simulink model "State_Flow_D"  (R2017a)
settings: Solver=FixedStepDiscrete  StartTime=0.0  StopTime=inf  FixedStep=0.001  RelTol=1e-3  EnableMultiTasking=on
libraries: xpcethercatlib x35, simulink x11, commutil2 x2
(part 2 of 3)

== system State_Flow_D/Out asse B Vite/Fungo ==
  In1 : Inport
  Constant : Constant  Value=0
  Data Type Conversion14 : DataTypeConversion
  Display10 : Display
  EtherCAT PDO Receive9 : xpcethercatlib/EtherCAT PDO Receive  Priority=2  sig_name=Beckoff.Channel 1.Input  sig_offset=0  sig_type=boolean  type_size=1  sig_dim=1  device_id=0  sample_time=0.001000
      settings: SourceProductName=Simulink Real-Time  SourceProductBaseCode=XP
  MATLAB Function : MATLAB Function  TreatAsAtomicUnit=on
  Memory : Memory
  Switch1 : Switch  Criteria=u2 ~= 0  Threshold=2
  Out1 : Outport
  wires:
  EtherCAT PDO Receive9/1 -> Data Type Conversion14/1
  Data Type Conversion14/1 -> MATLAB Function/2(old), Display10/1
  MATLAB Function/1(y) -> Memory/1
  In1/1 -> Switch1/3
  Memory/1 -> Switch1/2, MATLAB Function/1(now)
  Constant/1 -> Switch1/1
  Switch1/1 -> Out1/1

== system State_Flow_D/Sistema Braccia Linea/Velocita vite  ==
  EtherCAT PDO Receive14 : xpcethercatlib/EtherCAT PDO Receive  Priority=2  sig_name=AZ1.Transmit PDO 1.Axis A Actual motor velocity  sig_offset=48  sig_type=int32  type_size=32  sig_dim=1  device_id=0  sample_time=0.001000
      settings: SourceProductName=Simulink Real-Time  SourceProductBaseCode=XP
  EtherCAT PDO Receive15 : xpcethercatlib/EtherCAT PDO Receive  Priority=2  sig_name=AZ1.Transmit PDO 2.Axis B Actual motor velocity  sig_offset=136  sig_type=int32  type_size=32  sig_dim=1  device_id=0  sample_time=0.001000
      settings: SourceProductName=Simulink Real-Time  SourceProductBaseCode=XP
  Vel Asse A conv : MATLAB Function  TreatAsAtomicUnit=on
  Vel Asse B conv : MATLAB Function  TreatAsAtomicUnit=on
  Velocity A : DataTypeConversion
  Velocity B : DataTypeConversion
  Asse A : Outport
  Asse B : Outport  Port=2
  wires:
  EtherCAT PDO Receive15/1 -> Velocity B/1
  EtherCAT PDO Receive14/1 -> Velocity A/1
  Vel Asse A conv/1(vel_A_conv) -> Asse A/1
  Velocity B/1 -> Vel Asse B conv/1(p)
  Vel Asse B conv/1(vel_B_conv) -> Asse B/1
  Velocity A/1 -> Vel Asse A conv/1(vA)

== system State_Flow_D/Sistema Vite/Actual A ==
  Pos : Inport
  Offset : Inport  Port=2
  Rif asse B : Inport  Port=3
  Discrete Derivative A : simulink/Discrete/Discrete Derivative  gainval=1.0  ICPrevScaledInput=0.0  OutMin=[]  OutMax=[]  OutDataType=fixdt(1, 16)  OutScaling=2^-10  DoSatur=off
  Display31 : Display
  Posizione attuale Vite A : Subsystem
  Sum : Sum  Inputs=|-+
  A attuale : Outport
  wires:
  Offset/1 -> Sum/1
  Posizione attuale Vite A/1(A Att) -> A attuale/1, Discrete Derivative A/1
  Sum/1 -> Posizione attuale Vite A/1(Comp Vite A)
  Rif asse B/1 -> Posizione attuale Vite A/2("Comp Vite B ")
  Pos/1 -> Sum/2
  Discrete Derivative A/1 -> Display31/1

== system State_Flow_D/Sistema Vite/Clock reale ==
  cr : Inport
  offset : Inport  Port=2
  Sum2 : Sum  Inputs=-+|
  Ck : Outport
  wires:
  Sum2/1 -> Ck/1
  offset/1 -> Sum2/1
  cr/1 -> Sum2/2

== system State_Flow_D/Sistema Vite/Coppia VIte A finale ==
  Pos : Inport
  Vel : Inport  Port=2
  Gain : Gain  Gain=300*1000/0.36
  Gain6 : Gain  Gain=7.5*1000/0.36
  Sum9 : Sum  Inputs=|++
  Coppia : Outport
  wires:
  Pos/1 -> Gain/1
  Sum9/1 -> Coppia/1
  Gain6/1 -> Sum9/2
  Vel/1 -> Gain6/1
  Gain/1 -> Sum9/1

== system State_Flow_D/Sistema Vite/Velocita vite  ==
  EtherCAT PDO Receive14 : xpcethercatlib/EtherCAT PDO Receive  Priority=2  sig_name=AZ2.Transmit PDO 1.Axis A Actual motor velocity  sig_offset=304  sig_type=int32  type_size=32  sig_dim=1  device_id=0  sample_time=0.001000
      settings: SourceProductName=Simulink Real-Time  SourceProductBaseCode=XP
  EtherCAT PDO Receive15 : xpcethercatlib/EtherCAT PDO Receive  Priority=2  sig_name=AZ2.Transmit PDO 2.Axis B Actual motor velocity  sig_offset=392  sig_type=int32  type_size=32  sig_dim=1  device_id=0  sample_time=0.001000
      settings: SourceProductName=Simulink Real-Time  SourceProductBaseCode=XP
  Vel Asse A conv : MATLAB Function  TreatAsAtomicUnit=on
  Vel Asse B conv : MATLAB Function  TreatAsAtomicUnit=on
  Velocity A : DataTypeConversion
  Velocity B : DataTypeConversion
  Asse A : Outport
  Asse B : Outport  Port=2
  wires:
  EtherCAT PDO Receive15/1 -> Velocity B/1
  EtherCAT PDO Receive14/1 -> Velocity A/1
  Vel Asse A conv/1(vel_A_conv) -> Asse A/1
  Velocity B/1 -> Vel Asse B conv/1(p), Vel Asse A conv/2(vB)
  Vel Asse B conv/1(vel_B_conv) -> Asse B/1
  Velocity A/1 -> Vel Asse A conv/1(vA)

== system State_Flow_D/Sistema Vite/Actual A/Posizione attuale Vite A ==
  Comp Vite A : Inport
  "Comp Vite B " : Inport  Port=2
  Asse A conv : MATLAB Function  TreatAsAtomicUnit=on
  Asse B conv v : MATLAB Function  TreatAsAtomicUnit=on
  Sum5 : Sum
  A Att : Outport
  wires:
  Asse A conv/1(pos_A_conv) -> Sum5/1
  Asse B conv v/1(pos_B_conv_v) -> Sum5/2
  Comp Vite A/1 -> Asse A conv/1(p)
  Sum5/1 -> A Att/1
  "Comp Vite B "/1 -> Asse B conv v/1(p)

== matlab function State_Flow_D/Movimento Braccia/Cinematica Inversa1 ==
  data: x0old input; y0old input; theta1_0 input; theta2_0 input; time input; x0 output; y0 output
function [x0, y0] = fcn(x0old, y0old, theta1_0, theta2_0, time)

if time == 0 

d = 0.09; 
l = 0.25;

A = l^2*(sin(theta2_0)-sin(theta1_0))^2 + (-2*d -l*(cos(theta2_0)-cos(theta1_0)))^2;
B = -2*l^2*d*(sin(theta2_0)-sin(theta1_0))*(cos(theta2_0)+cos(theta1_0)) + ...
    l*(sin(theta2_0)-sin(theta1_0))*(-2*d -l*(cos(theta2_0)-cos(theta1_0)))*(-2*d -2*l*cos(theta2_0)) - ...
    2*l*sin(theta2_0)*(-2*d -l*(cos(theta2_0)-cos(theta1_0)))^2;
C = l^2*d^2*(cos(theta2_0)+cos(theta1_0))^2 -l*d*(cos(theta2_0)+cos(theta1_0))*(-2*d -l*(cos(theta2_0)-cos(theta1_0)))*(-2*d -2*l*cos(theta2_0)) + ...
    (d^2 + 2*d*l*cos(theta2_0))*(-2*d - l*(cos(theta2_0)-cos(theta1_0)))^2;

% Posizione Y end-effector
y0 = (-B + sqrt(B^2 - 4*A*C))/(2*A);
% Posizione X end-effector
x0 = (y0*l*(sin(theta2_0)-sin(theta1_0)) - l*d*(cos(theta2_0)+cos(theta1_0)))/(-2*d -l*(cos(theta2_0)-cos(theta1_0)));
else 
    x0 = x0old;
    y0 = y0old;
end

== matlab function State_Flow_D/Movimento Braccia/MATLAB Function ==
  data: x input; xp output; y input; yp output; bool input
function [xp,yp] = fcn(x, y, bool)
if bool == 4
    xp = x;
    yp = y;
else
    xp = 0;
    yp = 0;
end

== matlab function State_Flow_D/Sistema Braccia Linea/Velocita vite /Vel Asse A conv ==
  data: vA input; vel_A_conv output
function vel_A_conv = fcn(vA)
vel_A_conv = (vA)  *(2*pi)/163840/64;

== matlab function State_Flow_D/Sistema Braccia Linea/Velocita vite /Vel Asse B conv ==
  data: p input; vel_B_conv output
function vel_B_conv = fcn(p)
vel_B_conv = p  *(2*pi)/163840/64;

== matlab function State_Flow_D/Sistema Vite/Actual A/Posizione attuale Vite A/Asse A conv ==
  data: p input; pos_A_conv output
function pos_A_conv = fcn(p)
pos_A_conv = p * 0.02/(2*pi) * pi/2048/40;

== matlab function State_Flow_D/Sistema Vite/Rifermento Asse A Vite ==
  data: t input; ldm_pos output; h input; T input; ldm_vel output
function [ldm_pos, ldm_vel] = fcn(t,h,T)

xv = 0.3;
 x = t/T;
Ca=1/(xv*(1-xv));
Cv = 1/(1-xv);

if( x>= 0 && x < xv)
    f = Ca;
    F = Ca*x;
    G= Ca*x^2/2;
elseif(x >= xv && x < (1-xv) )
    f = 0;
    F = Cv;
    G= Ca*xv^2/2 + Cv*(x-xv);
elseif( x >= (1-xv) && x <= 1 )
    f = -Ca;
    xloc = x-(1-xv);
    F = Cv -Ca*xloc;
    G= Ca*xv^2/2 + Cv*(1-2*xv) + Cv*xloc -Ca*xloc^2/2;
else
    f=0;
    F=0;
    G= Ca*xv^2/2 + Cv*(1-2*xv) + Cv*xv -Ca*xv^2/2;
end

ldm_pos = G*h;
ldm_vel = F*h/T;

== matlab function State_Flow_D/LED Status/MATLAB Function ==
  data: u input; y output
function y = fcn(u)
if u == 2 ||u == 3
    y = 1;
else
    y = 0;
end

== matlab function State_Flow_D/LED Status/MATLAB Function1 ==
  data: u input; y output
function y = fcn(u)
if u == 1 || u == 2 || u == 4
    y = 1;
else
    y = 0;
end

== matlab function State_Flow_D/LED Status/MATLAB Function2 ==
  data: u input; y output
function y = fcn(u)
if u == 4 || u == 5
    y = 1;
else
    y = 0;
end

== matlab function State_Flow_D/Sistema Vite/Asse B conv ==
  data: p input; pos_B_conv output
function pos_B_conv = fcn(p)
pos_B_conv = p * pi/2048/40;

== matlab function State_Flow_D/Sistema Vite/Asse B ==
  data: t input; ldm_pos output; h input; T input; ldm_vel output
function [ldm_pos, ldm_vel] = fcn(t,h,T)

xv = 0.3;
 x = t/T;
Ca=1/(xv*(1-xv));
Cv = 1/(1-xv);

if( x>= 0 && x < xv)
    f = Ca;
    F = Ca*x;
    G= Ca*x^2/2;
elseif(x >= xv && x < (1-xv) )
    f = 0;
    F = Cv;
    G= Ca*xv^2/2 + Cv*(x-xv);
elseif( x >= (1-xv) && x <= 1 )
    f = -Ca;
    xloc = x-(1-xv);
    F = Cv -Ca*xloc;
    G= Ca*xv^2/2 + Cv*(1-2*xv) + Cv*xloc -Ca*xloc^2/2;
else
    f=0;
    F=0;
    G= Ca*xv^2/2 + Cv*(1-2*xv) + Cv*xv -Ca*xv^2/2;
end

ldm_pos = G*h;
ldm_vel = F*h/T;

== matlab function State_Flow_D/Sistema Vite/Actual A/Posizione attuale Vite A/Asse B conv v ==
  data: p input; pos_B_conv_v output
function pos_B_conv_v = fcn(p)
pos_B_conv_v = p * 0.02/(2*pi) * pi/2048/40;

== matlab function State_Flow_D/Sistema Vite/Velocita vite /Vel Asse A conv ==
  data: vA input; vel_A_conv output; vB input
function vel_A_conv = fcn(vA, vB)
vel_A_conv = (vA+vB) * 0.02/(2*pi) * pi/20480/40;

== matlab function State_Flow_D/Sistema Vite/Velocita vite /Vel Asse B conv ==
  data: p input; vel_B_conv output
function vel_B_conv = fcn(p)
vel_B_conv = p  * pi/20480/40;

== stateflow chart State_Flow_D/State flow robot ==
  settings: sampleTime=0.001
  state Step1
    entry:
    Bool = 0;
  state Step2
    entry:
    CoppiaH = 0;
  state Posizionamento
    state OffSet
      entry:
      CoppiaH = 0;
      CoppiaA = 0;
      CoppiaB = 0;
      OffA = posA;
      OffB = posB;
      OffA_0 = posA;
      OffB_0 = posB;
      Bool = 2;
      Luci = 3;
    state SetA
      entry:
      CoppiaA = 0;
      C1 = 0;
    state SetB1
      entry:
      CoppiaB = 0;
      C2 = 0;
    state Discesa_Vite
      entry:
      OffA_vite = posA_vite;
      CoppiaH=700;
    state SetB
      entry:
      CoppiaB = 0;
      C2 = 0;
    state SetA1
      entry:
      CoppiaA = 0;
      C1 = 0;
    Discesa_Vite -> OffSet : [posA_vite - OffA_vite >= 0.038/conv_vite]
    SetB1 -> Discesa_Vite : [C2 == 0]
    SetA -> SetB1 : [posB - OffB_0 >= 40*pi/180/conv]
    SetA1 -> Discesa_Vite : [C1 == 0]
    SetB -> SetA1 : [posA - OffA_0 >= 110*pi/180/conv]
  state Traiettoria
    entry:
    OffT = Clock;
    OffA_vite = posA_vite;
    OffB_vite = posB_vite;
    Luci = 4;
    Bool = 4;
  state Stop
    entry:
    Bool = 5;
    Luci = 5;
  state Coppie
    entry:
    OffA_0 = posA;
    OffB_0 = posB;
    CoppiaA = 1250;
    CoppiaB = 1250;
    CoppiaH = 0;
    Luci = 2;
  state Home
    entry:
    [CoppiaA, CoppiaB, CoppiaH] = Homing(fc, fcA, fcB);
    Bool = 1;
    conv =  (2*pi)/16384/64;
    conv_vite = 0.02/(2*pi) * pi/2048/40;
    Luci = 1;
    C1 = 1;
    C2 = 1;
    H = 0;
  state Step3
    entry:
    CoppiaA = 0;
    CoppiaB = 0;
  state [CA,CB,CH] = Homing(fc,fcA,fcB) [function]
  (default) -> Step1
  Coppie -> SetA [order 1] : [posA - OffA_0 >= 110*pi/180/conv]
  Step1 -> Home : [Status==1079]
  Step2 -> Coppie : [fcA == 1 && fcB==1]
  Home -> Step2 [order 2] : [fc==0]
  Traiettoria -> Stop : after(60,sec)
  OffSet -> Traiettoria
  Coppie -> SetB [order 2] : [posB - OffB_0 >= 40*pi/180/conv]
  Step3 -> Coppie : [fc==0]
  Home -> Step3 [order 1] : [fcA==1 && fcB==1]
  data: fc function_input double size=1; CA function_output; CB function_output; CH function_output; fcA function_input double size=1; fcB function_input double size=1; Clock input; posA_vite input; posB_vite input; SampleTime constant double; Status input; fc input; posA input; posB input; Bool output; OffT output; CoppiaH output; OffA_vite output; OffB_vite output; OffA output; OffB output; CoppiaA output; CoppiaB output; fcA input; fcB input; conv local; Luci output; OffA_0 local; OffB_0 local; C1 local; C2 local; conv_vite local; velA input; velB input; H output

== matlab function State_Flow_D/Movimento Braccia/Cinematica Inversa ==
  data: x input; theta1 output; y input; theta2 output
function [theta1, theta2] = fcn(x, y)

d = 0.09; 
l = 0.25;

p = 2*d*l + 2*x*l;
e = 2*y*l;
f = x^2 + d^2 + y^2 + 2*x*d;
a = -2*d*l + 2*x*l;
b = +2*y*l;
c = x^2 + d^2 + y^2 - 2*x*d;



   theta1 = 2*atan2(e + sqrt(p^2 + e^2 -f^2), p +f);


   theta2 = 2*atan2(b - sqrt(a^2 + b^2 -c^2), a +c);
   if (theta2) < -deg2rad(200)
       theta2 = theta2 + 2*pi;
   end

== matlab function State_Flow_D/Movimento Braccia/Asse B conv brac1 ==
  data: p input; pos_B_conv output
function pos_B_conv = fcn(p)
pos_B_conv = p * (2*pi)/16384/64;

== matlab function State_Flow_D/State flow robot/Homing/MATLAB Function ==
  data: fc input; CA output; fcA input; fcB input; CB output; CH output
function [CA, CB, CH] = fcn(fc, fcA, fcB)

CA = -1250;
CB = -1250;
CH = -600;

if fc < 1
    CH = 0;
end
if fcA == 1
    CA = 0;
end
if fcB == 1
    CB = 0;
end

== matlab function State_Flow_D/Out asse A Vite/Fungo/MATLAB Function ==
  data: now input; old input; y output
function y = fcn(now, old)
if old == 0 && now == 1
    y = 1;
else
    y = old;
end

== matlab function State_Flow_D/Out asse B Vite/Fungo/MATLAB Function ==
  data: now input; old input; y output
function y = fcn(now, old)
if old == 0 && now == 1
    y = 1;
else
    y = old;
end

== matlab function State_Flow_D/Out Asse A Braccia/Fungo/MATLAB Function ==
  data: now input; old input; y output
function y = fcn(now, old)
if old == 0 && now == 1
    y = 1;
else
    y = old;
end

== matlab function State_Flow_D/Out Asse B Braccia/Fungo/MATLAB Function ==
  data: now input; old input; y output
function y = fcn(now, old)
if old == 0 && now == 1
    y = 1;
else
    y = old;
end

== matlab function State_Flow_D/Velocita vite /Vel Asse A conv ==
  data: vA input; vel_A_conv output
function vel_A_conv = fcn(vA)
vel_A_conv = (vA)  *(2*pi)/163840/64;

== matlab function State_Flow_D/Velocita vite /Vel Asse B conv ==
  data: p input; vel_B_conv output
function vel_B_conv = fcn(p)
vel_B_conv = p  *(2*pi)/163840/64;

== matlab function State_Flow_D/Sistema Braccia Linea/Asse A conv bracc2 ==
  data: p input; pos_A_conv output
function pos_A_conv = fcn(p)
pos_A_conv = p * (2*pi)/16384/64;

== matlab function State_Flow_D/Sistema Braccia Linea/Asse B conv brac1 ==
  data: p input; pos_B_conv output
function pos_B_conv = fcn(p)
pos_B_conv = p * (2*pi)/16384/64;

== matlab function State_Flow_D/Sistema Braccia Linea/Cinematica Inversa ==
  data: x input; theta1 output; y input; theta2 output
function [theta1, theta2] = fcn(x, y)

d = 0.09; 
l = 0.25;

p = 2*d*l + 2*x*l;
e = 2*y*l;
f = x^2 + d^2 + y^2 + 2*x*d;
a = -2*d*l + 2*x*l;
b = +2*y*l;
c = x^2 + d^2 + y^2 - 2*x*d;



   theta1 = 2*atan2(e + sqrt(p^2 + e^2 -f^2), p +f);


   theta2 = 2*atan2(b - sqrt(a^2 + b^2 -c^2), a +c);
   if (theta2) < -deg2rad(200)
       theta2 = theta2 + 2*pi;
   end

== matlab function State_Flow_D/Sistema Braccia Linea/Cinematica Inversa vel ==
  data: theta1 input; theta2 input; x input; y input; xp input; theta1_p output; yp input; theta2_p output
function [theta1_p, theta2_p] = fcn(theta1, theta2,x, y, xp, yp)

d = 0.09; 
l = 0.25;

N21 = -l*sin(theta1)*(x+d-l*cos(theta1)) + l*cos(theta1)*(y-l*sin(theta1));

N22 = -l*cos(theta2)*(y-l*sin(theta2))*(x+d-l*cos(theta1))/(x-d-l*cos(theta2)) + l*sin(theta2)*(x+d-l*cos(theta1));

D2 = y-l*sin(theta1) - (y-l*sin(theta2))*(x+d-l*cos(theta1))/(x-d-l*cos(theta2));

J21 = N21/D2;

J22 = N22/D2;

J11 = -(y-l*sin(theta2))/(x-d-l*cos(theta2))*(J21);

J12 = -(y-l*sin(theta2))/(x-d-l*cos(theta2))*(J22) -l*sin(theta2) + (y-l*sin(theta2))/(x-d-l*cos(theta2))*(l*cos(theta2));

J = [J11 J12; J21 J22];

theta_p = J^-1 * [xp; yp];
theta1_p = theta_p(1);
theta2_p = theta_p(2);

== matlab function State_Flow_D/Sistema Braccia Linea/Cinematica Inversa1 ==
  data: theta1_0 input; x0 output; theta2_0 input; y0 output
function [x0, y0] = fcn(theta1_0, theta2_0)

d = 0.09; 
l = 0.25;

A = l^2*(sin(theta2_0)-sin(theta1_0))^2 + (-2*d -l*(cos(theta2_0)-cos(theta1_0)))^2;
B = -2*l^2*d*(sin(theta2_0)-sin(theta1_0))*(cos(theta2_0)+cos(theta1_0)) + ...
    l*(sin(theta2_0)-sin(theta1_0))*(-2*d -l*(cos(theta2_0)-cos(theta1_0)))*(-2*d -2*l*cos(theta2_0)) - ...
    2*l*sin(theta2_0)*(-2*d -l*(cos(theta2_0)-cos(theta1_0)))^2;
C = l^2*d^2*(cos(theta2_0)+cos(theta1_0))^2 -l*d*(cos(theta2_0)+cos(theta1_0))*(-2*d -l*(cos(theta2_0)-cos(theta1_0)))*(-2*d -2*l*cos(theta2_0)) + ...
    (d^2 + 2*d*l*cos(theta2_0))*(-2*d - l*(cos(theta2_0)-cos(theta1_0)))^2;

% Posizione Y end-effector
y0 = (-B + sqrt(B^2 - 4*A*C))/(2*A)
% Posizione X end-effector
x0 = (y0*l*(sin(theta2_0)-sin(theta1_0)) - l*d*(cos(theta2_0)+cos(theta1_0)))/(-2*d -l*(cos(theta2_0)-cos(theta1_0)))

== matlab function State_Flow_D/Sistema Braccia Linea/x ==
  data: t input; ldm_pos output; h input; T input; ldm_vel output
function [ldm_pos, ldm_vel] = fcn(t,h,T)

xv = 0.3;
 x = t/T;
Ca=1/(xv*(1-xv));
Cv = 1/(1-xv);

if( x>= 0 && x < xv)
    f = Ca;
    F = Ca*x;
    G= Ca*x^2/2;
elseif(x >= xv && x < (1-xv) )
    f = 0;
    F = Cv;
    G= Ca*xv^2/2 + Cv*(x-xv);
elseif( x >= (1-xv) && x <= 1 )
    f = -Ca;
    xloc = x-(1-xv);
    F = Cv -Ca*xloc;
    G= Ca*xv^2/2 + Cv*(1-2*xv) + Cv*xloc -Ca*xloc^2/2;
else
    f=0;
    F=0;
    G= Ca*xv^2/2 + Cv*(1-2*xv) + Cv*xv -Ca*xv^2/2;
end

ldm_pos = G*h;
ldm_vel = F*h/T;

== matlab function State_Flow_D/Sistema Braccia Linea/y ==
  data: t input; ldm_pos output; h input; T input; ldm_vel output
function [ldm_pos, ldm_vel] = fcn(t,h,T)

xv = 0.3;
 x = t/T;
Ca=1/(xv*(1-xv));
Cv = 1/(1-xv);

if( x>= 0 && x < xv)
    f = Ca;
    F = Ca*x;
    G= Ca*x^2/2;
elseif(x >= xv && x < (1-xv) )
    f = 0;
    F = Cv;
    G= Ca*xv^2/2 + Cv*(x-xv);
elseif( x >= (1-xv) && x <= 1 )
    f = -Ca;
    xloc = x-(1-xv);
    F = Cv -Ca*xloc;
    G= Ca*xv^2/2 + Cv*(1-2*xv) + Cv*xloc -Ca*xloc^2/2;
else
    f=0;
    F=0;
    G= 1;
end

ldm_pos = G*h;
ldm_vel = F*h/T;

== matlab function State_Flow_D/Movimento Braccia/Asse A conv brac ==
  data: p input; pos_A_conv output
function pos_A_conv = fcn(p)
pos_A_conv = p * (2*pi)/16384/64;

== matlab function State_Flow_D/Movimento Braccia/Subsystem/Cerchio ==
  data: xc output; t input; yc output; T input; r input; xc_p output; yc_p output
function [xc, yc, xc_p, yc_p] = fcn(t, T, r)
xv = 0.4;
xj = 0.1;
x = t/T;
Ca = 1/((1-xv)*(xv-xj));
if ( x >= 0 && x < xj)            %acc crescente positiva
    f = Ca/xj*x;
    F = (1/2)*Ca/xj*x^2;
    G = (1/6)*Ca/xj*x^3;
    J = Ca/xj;

  elseif (x >= xj && x < (xv-xj))   %acc costante positiva
    f = Ca;
    F = Ca*x - (1/2)*Ca*xj;
    G = (1/2)*Ca*x^2 - (1/2)*Ca*xj*x + (1/6)*Ca*xj^2;
    J = 0;

  elseif( x>= (xv-xj) && x < xv)    %acc decrescente positiva
    f = -Ca/xj*x + Ca*xv/xj;
    F = -(1/2)*Ca/xj*x^2 + Ca/xj*xv*x - Ca*(xj + (1/2)/xj*xv^2 - xv);
    G = -(1/6)*Ca/xj*x^3 + (1/2)*Ca/xj*xv*x^2 - Ca*(xj + (1/2)/xj*xv^2 - xv)*x ...
        - (1/2)*Ca*xv^2  + (1/6)*Ca/xj*xv^3 + (1/2)*Ca*xv*xj;
    J = -Ca/xj;

  elseif( x>= xv && x < (1-xv))     %acc costante nulla
    f = 0;
    F = Ca*(xv - xj);
    G = Ca*(xv - xj)*x - (1/2)*Ca*xv^2 + (1/2)*Ca*xv*xj;
    J = 0;
    
  elseif( x>= (1-xv) && x < (1-xv+xj))   %acc decrescente negativa
    f = -Ca/xj*x + Ca/xj*(1-xv);
    F = -(1/2)*Ca/xj*x^2 + Ca/xj*(1-xv)*x + Ca*(xv-xj) - (1/2)*Ca/xj*(1-xv)^2;
    G = -(1/6)*Ca/xj*x^3 + (1/2)*Ca/xj*(1-xv)*x^2 + Ca*(xv-xj)*x - (1/2)*Ca/xj*(1-xv)^2*x ...
        - (1/2)*Ca*xv^2 + (1/2)*Ca*xv*xj + (1/6)*Ca/xj*(1-xv)^3;
    J = -Ca/xj;
    
  elseif( x>= (1-xv+xj) && x < (1-xj))   %acc costante negativa
    f = -Ca; 
    F = -Ca*x + Ca - (1/2)*Ca*xj;
    G = -(1/2)*Ca*x^2 + Ca*x - (1/2)*Ca*xj*x + 1 - Ca*(-(1/2)*xj + (1/6)*xj^2 + (1/2));
    J = 0;
    
  elseif( x>= (1-xj) && x <= 1)          %acc crescente negativa
    f = Ca/xj*(x-1);
    F = (1/2)*Ca/xj*x^2 - Ca/xj*x +(1/2)*Ca/xj;
    G = (1/6)*Ca/xj*x^3 - (1/2)*Ca/xj*x^2 +(1/2)*Ca/xj*x + 1 - (1/6)*Ca/xj;
    J = Ca/xj;
    
  else                                   %acc costante nulla
    f = 0;
    F = 0;
    G = 1;
    J = 0;
end
  
 alfa = G*2*pi;
 alfa_p = F*2*pi/T;
 xc = r*cos(pi/2-alfa);
 yc = r*sin(pi/2-alfa) - r;
 xc_p = r*sin(pi/2-alfa)*alfa_p;
 yc_p = -r*cos(pi/2-alfa)*alfa_p;

== matlab function State_Flow_D/Movimento Braccia/Subsystem/Quadrato ==
  data: xq output; yq output; t input; T input; h input; xq_p output; yq_p output
function [xq, yq, xq_p, yq_p] = fcn(t, T, h)
xv = 0.4;
xj = 0.1;
x1 = t/(0.5*T/4);
x2 = (t-0.5*T/4)/(T/4);
x3 = (t-1.5*T/4)/(T/4);
x4 = (t-2.5*T/4)/(T/4);
x5 = (t-3.5*T/4)/(0.5*T/4);
Ca = 1/((1-xv)*(xv-xj));
% Ca = 1/(xv*(1-xv));
% Cv = 1/(1-xv);


if t > 0 && t <= 0.5*T/4
  
  if ( x1 >= 0 && x1 < xj)            %acc crescente positiva
    f = Ca/xj*x1;
    F = (1/2)*Ca/xj*x1^2;
    G = (1/6)*Ca/xj*x1^3;
    J = Ca/xj;

  elseif (x1 >= xj && x1 < (xv-xj))   %acc costante positiva
    f = Ca;
    F = Ca*x1 - (1/2)*Ca*xj;
    G = (1/2)*Ca*x1^2 - (1/2)*Ca*xj*x1 + (1/6)*Ca*xj^2;
    J = 0;

  elseif( x1>= (xv-xj) && x1 < xv)    %acc decrescente positiva
    f = -Ca/xj*x1 + Ca*xv/xj;
    F = -(1/2)*Ca/xj*x1^2 + Ca/xj*xv*x1 - Ca*(xj + (1/2)/xj*xv^2 - xv);
    G = -(1/6)*Ca/xj*x1^3 + (1/2)*Ca/xj*xv*x1^2 - Ca*(xj + (1/2)/xj*xv^2 - xv)*x1 ...
        - (1/2)*Ca*xv^2  + (1/6)*Ca/xj*xv^3 + (1/2)*Ca*xv*xj;
    J = -Ca/xj;

  elseif( x1>= xv && x1 < (1-xv))     %acc costante nulla
    f = 0;
    F = Ca*(xv - xj);
    G = Ca*(xv - xj)*x1 - (1/2)*Ca*xv^2 + (1/2)*Ca*xv*xj;
    J = 0;
    
  elseif( x1>= (1-xv) && x1 < (1-xv+xj))   %acc decrescente negativa
    f = -Ca/xj*x1 + Ca/xj*(1-xv);
    F = -(1/2)*Ca/xj*x1^2 + Ca/xj*(1-xv)*x1 + Ca*(xv-xj) - (1/2)*Ca/xj*(1-xv)^2;
    G = -(1/6)*Ca/xj*x1^3 + (1/2)*Ca/xj*(1-xv)*x1^2 + Ca*(xv-xj)*x1 - (1/2)*Ca/xj*(1-xv)^2*x1 ...
        - (1/2)*Ca*xv^2 + (1/2)*Ca*xv*xj + (1/6)*Ca/xj*(1-xv)^3;
    J = -Ca/xj;
    
  elseif( x1>= (1-xv+xj) && x1 < (1-xj))   %acc costante negativa
    f = -Ca; 
    F = -Ca*x1 + Ca - (1/2)*Ca*xj;
    G = -(1/2)*Ca*x1^2 + Ca*x1 - (1/2)*Ca*xj*x1 + 1 - Ca*(-(1/2)*xj + (1/6)*xj^2 + (1/2));
    J = 0;
    
  elseif( x1>= (1-xj) && x1 <= 1)          %acc crescente negativa
    f = Ca/xj*(x1-1);
    F = (1/2)*Ca/xj*x1^2 - Ca/xj*x1 +(1/2)*Ca/xj;
    G = (1/6)*Ca/xj*x1^3 - (1/2)*Ca/xj*x1^2 +(1/2)*Ca/xj*x1 + 1 - (1/6)*Ca/xj;
    J = Ca/xj;
    
  else                                   %acc costante nulla
    f = 0;
    F = 0;
    G = 1;
    J = 0;
  end
    xq = G*h/2;
    xq_p = F*(h/2)/(T/4);
    yq = 0;
    yq_p = 0; 

elseif t > 0.5*T/4 && t <= 1.5*T/4
    Ca = 1/((1-xv)*(xv-xj));
% Cj = Ca/xj;
  
  if ( x2 >= 0 && x2 < xj)            %acc crescente positiva
    f = Ca/xj*x2;
    F = (1/2)*Ca/xj*x2^2;
    G = (1/6)*Ca/xj*x2^3;
    J = Ca/xj;

  elseif (x2 >= xj && x2 < (xv-xj))   %acc costante positiva
    f = Ca;
    F = Ca*x2 - (1/2)*Ca*xj;
    G = (1/2)*Ca*x2^2 - (1/2)*Ca*xj*x2 + (1/6)*Ca*xj^2;
    J = 0;

  elseif( x2>= (xv-xj) && x2 < xv)    %acc decrescente positiva
    f = -Ca/xj*x2 + Ca*xv/xj;
    F = -(1/2)*Ca/xj*x2^2 + Ca/xj*xv*x2 - Ca*(xj + (1/2)/xj*xv^2 - xv);
    G = -(1/6)*Ca/xj*x2^3 + (1/2)*Ca/xj*xv*x2^2 - Ca*(xj + (1/2)/xj*xv^2 - xv)*x2 ...
        - (1/2)*Ca*xv^2  + (1/6)*Ca/xj*xv^3 + (1/2)*Ca*xv*xj;
    J = -Ca/xj;

  elseif( x2>= xv && x2 < (1-xv))     %acc costante nulla
    f = 0;
    F = Ca*(xv - xj);
    G = Ca*(xv - xj)*x2 - (1/2)*Ca*xv^2 + (1/2)*Ca*xv*xj;
    J = 0;
    
  elseif( x2>= (1-xv) && x2 < (1-xv+xj))   %acc decrescente negativa
    f = -Ca/xj*x2 + Ca/xj*(1-xv);
    F = -(1/2)*Ca/xj*x2^2 + Ca/xj*(1-xv)*x2 + Ca*(xv-xj) - (1/2)*Ca/xj*(1-xv)^2;
    G = -(1/6)*Ca/xj*x2^3 + (1/2)*Ca/xj*(1-xv)*x2^2 + Ca*(xv-xj)*x2 - (1/2)*Ca/xj*(1-xv)^2*x2 ...
        - (1/2)*Ca*xv^2 + (1/2)*Ca*xv*xj + (1/6)*Ca/xj*(1-xv)^3;
    J = -Ca/xj;
    
  elseif( x2>= (1-xv+xj) && x2 < (1-xj))   %acc costante negativa
    f = -Ca; 
    F = -Ca*x2 + Ca - (1/2)*Ca*xj;
    G = -(1/2)*Ca*x2^2 + Ca*x2 - (1/2)*Ca*xj*x2 + 1 - Ca*(-(1/2)*xj + (1/6)*xj^2 + (1/2));
    J = 0;
    
  elseif( x2>= (1-xj) && x2 <= 1)          %acc crescente negativa
    f = Ca/xj*(x2-1);
    F = (1/2)*Ca/xj*x2^2 - Ca/xj*x2 +(1/2)*Ca/xj;
    G = (1/6)*Ca/xj*x2^3 - (1/2)*Ca/xj*x2^2 +(1/2)*Ca/xj*x2 + 1 - (1/6)*Ca/xj;
    J = Ca/xj;
    
  else                                   %acc costante nulla
    f = 0;
    F = 0;
    G = 1;
    J = 0;
  end
    xq = h/2;
    xq_p = 0;
    yq = -G*h; 
    yq_p = -F*h/(T/4); 

elseif t > 1.5*T/4 && t <= 2.5*T/4
     Ca = 1/((1-xv)*(xv-xj));
% Cj = Ca/xj;
  
  if ( x3 >= 0 && x3 < xj)            %acc crescente positiva
    f = Ca/xj*x3;
    F = (1/2)*Ca/xj*x3^2;
    G = (1/6)*Ca/xj*x3^3;
    J = Ca/xj;

  elseif (x3 >= xj && x3 < (xv-xj))   %acc costante positiva
    f = Ca;
    F = Ca*x3 - (1/2)*Ca*xj;
    G = (1/2)*Ca*x3^2 - (1/2)*Ca*xj*x3 + (1/6)*Ca*xj^2;
    J = 0;

  elseif( x3>= (xv-xj) && x3 < xv)    %acc decrescente positiva
    f = -Ca/xj*x3 + Ca*xv/xj;
    F = -(1/2)*Ca/xj*x3^2 + Ca/xj*xv*x3 - Ca*(xj + (1/2)/xj*xv^2 - xv);
    G = -(1/6)*Ca/xj*x3^3 + (1/2)*Ca/xj*xv*x3^2 - Ca*(xj + (1/2)/xj*xv^2 - xv)*x3 ...
        - (1/2)*Ca*xv^2  + (1/6)*Ca/xj*xv^3 + (1/2)*Ca*xv*xj;
    J = -Ca/xj;

  elseif( x3>= xv && x3 < (1-xv))     %acc costante nulla
    f = 0;
    F = Ca*(xv - xj);
    G = Ca*(xv - xj)*x3 - (1/2)*Ca*xv^2 + (1/2)*Ca*xv*xj;
    J = 0;
    
  elseif( x3>= (1-xv) && x3 < (1-xv+xj))   %acc decrescente negativa
    f = -Ca/xj*x3 + Ca/xj*(1-xv);
    F = -(1/2)*Ca/xj*x3^2 + Ca/xj*(1-xv)*x3 + Ca*(xv-xj) - (1/2)*Ca/xj*(1-xv)^2;
    G = -(1/6)*Ca/xj*x3^3 + (1/2)*Ca/xj*(1-xv)*x3^2 + Ca*(xv-xj)*x3 - (1/2)*Ca/xj*(1-xv)^2*x3 ...
        - (1/2)*Ca*xv^2 + (1/2)*Ca*xv*xj + (1/6)*Ca/xj*(1-xv)^3;
    J = -Ca/xj;
    
  elseif( x3>= (1-xv+xj) && x3 < (1-xj))   %acc costante negativa
    f = -Ca; 
    F = -Ca*x3 + Ca - (1/2)*Ca*xj;
    G = -(1/2)*Ca*x3^2 + Ca*x3 - (1/2)*Ca*xj*x3 + 1 - Ca*(-(1/2)*xj + (1/6)*xj^2 + (1/2));
    J = 0;
    
  elseif( x3>= (1-xj) && x3 <= 1)          %acc crescente negativa
    f = Ca/xj*(x3-1);
    F = (1/2)*Ca/xj*x3^2 - Ca/xj*x3 +(1/2)*Ca/xj;
    G = (1/6)*Ca/xj*x3^3 - (1/2)*Ca/xj*x3^2 +(1/2)*Ca/xj*x3 + 1 - (1/6)*Ca/xj;
    J = Ca/xj;
    
  else                                   %acc costante nulla
    f = 0;
    F = 0;
    G = 1;
    J = 0;
  end
    xq = h/2-G*h;
    xq_p = -F*h/(T/4);
    yq = -h; 
    yq_p = 0; 
 
elseif t > 2.5*T/4 && t <= 3.5*T/4
   Ca = 1/((1-xv)*(xv-xj));
% Cj = Ca/xj;
  
  if ( x4 >= 0 && x4 < xj)            %acc crescente positiva
    f = Ca/xj*x4;
    F = (1/2)*Ca/xj*x4^2;
    G = (1/6)*Ca/xj*x4^3;
    J = Ca/xj;

  elseif (x4 >= xj && x4 < (xv-xj))   %acc costante positiva
    f = Ca;
    F = Ca*x4 - (1/2)*Ca*xj;
    G = (1/2)*Ca*x4^2 - (1/2)*Ca*xj*x4 + (1/6)*Ca*xj^2;
    J = 0;

  elseif( x4>= (xv-xj) && x4 < xv)    %acc decrescente positiva
    f = -Ca/xj*x4 + Ca*xv/xj;
    F = -(1/2)*Ca/xj*x4^2 + Ca/xj*xv*x4 - Ca*(xj + (1/2)/xj*xv^2 - xv);
    G = -(1/6)*Ca/xj*x4^3 + (1/2)*Ca/xj*xv*x4^2 - Ca*(xj + (1/2)/xj*xv^2 - xv)*x4 ...
        - (1/2)*Ca*xv^2  + (1/6)*Ca/xj*xv^3 + (1/2)*Ca*xv*xj;
    J = -Ca/xj;

  elseif( x4>= xv && x4 < (1-xv))     %acc costante nulla
    f = 0;
    F = Ca*(xv - xj);
    G = Ca*(xv - xj)*x4 - (1/2)*Ca*xv^2 + (1/2)*Ca*xv*xj;
    J = 0;
    
  elseif( x4>= (1-xv) && x4 < (1-xv+xj))   %acc decrescente negativa
    f = -Ca/xj*x4 + Ca/xj*(1-xv);
    F = -(1/2)*Ca/xj*x4^2 + Ca/xj*(1-xv)*x4 + Ca*(xv-xj) - (1/2)*Ca/xj*(1-xv)^2;
    G = -(1/6)*Ca/xj*x4^3 + (1/2)*Ca/xj*(1-xv)*x4^2 + Ca*(xv-xj)*x4 - (1/2)*Ca/xj*(1-xv)^2*x4 ...
        - (1/2)*Ca*xv^2 + (1/2)*Ca*xv*xj + (1/6)*Ca/xj*(1-xv)^3;
    J = -Ca/xj;
    
  elseif( x4>= (1-xv+xj) && x4 < (1-xj))   %acc costante negativa
    f = -Ca; 
    F = -Ca*x4 + Ca - (1/2)*Ca*xj;
    G = -(1/2)*Ca*x4^2 + Ca*x4 - (1/2)*Ca*xj*x4 + 1 - Ca*(-(1/2)*xj + (1/6)*xj^2 + (1/2));
    J = 0;
    
  elseif( x4>= (1-xj) && x4 <= 1)          %acc crescente negativa
    f = Ca/xj*(x4-1);
    F = (1/2)*Ca/xj*x4^2 - Ca/xj*x4 +(1/2)*Ca/xj;
    G = (1/6)*Ca/xj*x4^3 - (1/2)*Ca/xj*x4^2 +(1/2)*Ca/xj*x4 + 1 - (1/6)*Ca/xj;
    J = Ca/xj;
    
  else                                   %acc costante nulla
    f = 0;
    F = 0;
    G = 1;
    J = 0;
  end
    xq = -h/2;
    xq_p = 0;
    yq = -h + G*h;
    yq_p = F*h/(T/4); 

elseif t > 3.5*T/4 && t <= 4*T/4
   Ca = 1/((1-xv)*(xv-xj));
% Cj = Ca/xj;
  
  if ( x5 >= 0 && x5 < xj)            %acc crescente positiva
    f = Ca/xj*x5;
    F = (1/2)*Ca/xj*x5^2;
    G = (1/6)*Ca/xj*x5^3;
    J = Ca/xj;

  elseif (x5 >= xj && x5 < (xv-xj))   %acc costante positiva
    f = Ca;
    F = Ca*x5 - (1/2)*Ca*xj;
    G = (1/2)*Ca*x5^2 - (1/2)*Ca*xj*x5 + (1/6)*Ca*xj^2;
    J = 0;

  elseif( x5>= (xv-xj) && x5 < xv)    %acc decrescente positiva
    f = -Ca/xj*x5 + Ca*xv/xj;
    F = -(1/2)*Ca/xj*x5^2 + Ca/xj*xv*x5 - Ca*(xj + (1/2)/xj*xv^2 - xv);
    G = -(1/6)*Ca/xj*x5^3 + (1/2)*Ca/xj*xv*x5^2 - Ca*(xj + (1/2)/xj*xv^2 - xv)*x5 ...
        - (1/2)*Ca*xv^2  + (1/6)*Ca/xj*xv^3 + (1/2)*Ca*xv*xj;
    J = -Ca/xj;

  elseif( x5>= xv && x5 < (1-xv))     %acc costante nulla
    f = 0;
    F = Ca*(xv - xj);
    G = Ca*(xv - xj)*x5 - (1/2)*Ca*xv^2 + (1/2)*Ca*xv*xj;
    J = 0;
    
  elseif( x5>= (1-xv) && x5 < (1-xv+xj))   %acc decrescente negativa
    f = -Ca/xj*x5 + Ca/xj*(1-xv);
    F = -(1/2)*Ca/xj*x5^2 + Ca/xj*(1-xv)*x5 + Ca*(xv-xj) - (1/2)*Ca/xj*(1-xv)^2;
    G = -(1/6)*Ca/xj*x5^3 + (1/2)*Ca/xj*(1-xv)*x5^2 + Ca*(xv-xj)*x5 - (1/2)*Ca/xj*(1-xv)^2*x5 ...
        - (1/2)*Ca*xv^2 + (1/2)*Ca*xv*xj + (1/6)*Ca/xj*(1-xv)^3;
    J = -Ca/xj;
    
  elseif( x5>= (1-xv+xj) && x5 < (1-xj))   %acc costante negativa
    f = -Ca; 
    F = -Ca*x5 + Ca - (1/2)*Ca*xj;
    G = -(1/2)*Ca*x5^2 + Ca*x5 - (1/2)*Ca*xj*x5 + 1 - Ca*(-(1/2)*xj + (1/6)*xj^2 + (1/2));
    J = 0;
    
  elseif( x5>= (1-xj) && x5 <= 1)          %acc crescente negativa
    f = Ca/xj*(x5-1);
    F = (1/2)*Ca/xj*x5^2 - Ca/xj*x5 +(1/2)*Ca/xj;
    G = (1/6)*Ca/xj*x5^3 - (1/2)*Ca/xj*x5^2 +(1/2)*Ca/xj*x5 + 1 - (1/6)*Ca/xj;
    J = Ca/xj;
    
  else                                   %acc costante nulla
    f = 0;
    F = 0;
    G = 1;
    J = 0;
  end
    xq = -h/2 + G*h/2;
    xq_p = F*h/2/(T/4);
    yq = 0
    yq_p = 0; 
else
xq = 0;
yq = 0;
xq_p = 0;
yq_p = 0; 
end

== matlab function State_Flow_D/Movimento Braccia/Quadrato1 ==
  data: x output; t input; y output; T input; h input
function [x, y] = fcn(t, T, h)
X1 = linspace(0, h, 1000*T/4);
X2 = linspace(h, 0, 1000*T/4);
Y1 = linspace(0, -h, 1000*T/4);
Y2 = linspace(-h, 0, 1000*T/4);

if t > 0 && t <= T/4
    y = 0;
    x = X1(t*1000);
elseif t > T/4 && t <= 2*T/4
    x = h;
    y = Y1((t-T/4)*1000);
elseif t > 2*T/4 && t <= 3*T/4
    y = -h;
    x = X2((t-2*T/4)*1000);
elseif t > 3*T/4 && t <= 4*T/4
    x = 0;
    y = Y2((t-3*T/4)*1000);
else
x = 0;
y = 0;
end

== matlab function State_Flow_D/Movimento Braccia/Cinematica Inversa vel ==
  data: theta1 input; theta2 input; x input; y input; xp input; theta1_p output; yp input; theta2_p output
function [theta1_p, theta2_p] = fcn(theta1, theta2,x, y, xp, yp)

d = 0.09; 
l = 0.25;

N21 = -l*sin(theta1)*(x+d-l*cos(theta1)) + l*cos(theta1)*(y-l*sin(theta1));

N22 = -l*cos(theta2)*(y-l*sin(theta2))*(x+d-l*cos(theta1))/(x-d-l*cos(theta2)) + l*sin(theta2)*(x+d-l*cos(theta1));

D2 = y-l*sin(theta1) - (y-l*sin(theta2))*(x+d-l*cos(theta1))/(x-d-l*cos(theta2));

J21 = N21/D2;

J22 = N22/D2;

J11 = -(y-l*sin(theta2))/(x-d-l*cos(theta2))*(J21);

J12 = -(y-l*sin(theta2))/(x-d-l*cos(theta2))*(J22) -l*sin(theta2) + (y-l*sin(theta2))/(x-d-l*cos(theta2))*(l*cos(theta2));

J = [J11 J12; J21 J22];

theta_p = J^-1 * [xp; yp];
theta1_p = theta_p(1);
theta2_p = theta_p(2);

== matlab function State_Flow_D/Movimento Braccia/Velocita vite /Vel Asse A conv ==
  data: vA input; vel_A_conv output
function vel_A_conv = fcn(vA)
vel_A_conv = (vA)  *(2*pi)/163840/64;

== matlab function State_Flow_D/Movimento Braccia/Velocita vite /Vel Asse B conv ==
  data: p input; vel_B_conv output
function vel_B_conv = fcn(p)
vel_B_conv = p  *(2*pi)/163840/64;

== matlab function State_Flow_D/Movimento/MATLAB Function ==
  data: x input; xp output; y input; yp output; bool input
function [xp,yp] = fcn(x, y, bool)
if bool == 4
    xp = x;
    yp = y;
else
    xp = 0;
    yp = 0;
end

== matlab function State_Flow_D/Out Asse A Braccia/MATLAB Function ==
  data: C input; Cout output
function Cout = fcn(C)
if C >= 800 && C <= 1000
Cout = 1200;
elseif C >= 1700 && C <= 2000
Cout = 1500;
elseif C <= -800 && C >= -1000
Cout = -1200;
elseif C <= -1700 && C >= -2000
Cout = -1500; 
else 
Cout = C;
end

== matlab function State_Flow_D/Out Asse B Braccia/MATLAB Function ==
  data: C input; Cout output
function Cout = fcn(C)
if C >= 800 && C <= 1000
Cout = 1200;
elseif C >= 1700 && C <= 2000
Cout = 1500;
elseif C <= -800 && C >= -1000
Cout = -1200;
elseif C <= -1700 && C >= -2000
Cout = -1500; 
else 
Cout = C;
end

== matlab function State_Flow_D/Movimento Braccia/Subsystem/g ==
  data: x output; y output; x_p output; t input; l input; T input; y_p output
function [x, y, x_p,y_p] = fcn(t, l, T)
 Tt = T/32;
 t1 = (t-0*Tt/2)/(Tt/2);
 t2 = (t-1*Tt/2)/Tt;
 t3 = (t-3*Tt/2)/(Tt/2);
 t4 = (t-4*Tt/2)/(Tt/2);
 t5 = (t-5*Tt/2)/Tt;
 t6 = (t-7*Tt/2)/Tt;
 t7 = (t-9*Tt/2)/Tt;
 t8 = (t-11*Tt/2)/(Tt/2);
 t9 = (t-12*Tt/2)/(Tt/2);
 t10 = (t-13*Tt/2)/Tt;
 t11 = (t-15*Tt/2)/(Tt/2);
 t12 = (t-16*Tt/2)/(Tt/2);
 t13 = (t-17*Tt/2)/Tt;
 t14 = (t-19*Tt/2)/(Tt/2);
 t15 = (t-20*Tt/2)/(Tt/2);
 t16 = (t-21*Tt/2)/Tt;
 t17 = (t-23*Tt/2)/Tt;
 t18 = (t-25*Tt/2)/Tt;
 t19 = (t-27*Tt/2)/(Tt/2);
 t20 = (t-28*Tt/2)/(Tt/2);
 t21 = (t-29*Tt/2)/Tt;
 t22 = (t-31*Tt/2)/(Tt/2);
 t23 = (t-32*Tt/2)/(Tt/2);
 t24 = (t-33*Tt/2)/Tt;
 t25 = (t-35*Tt/2)/(Tt/2);
 t26 = (t-36*Tt/2)/(Tt/2);
 t27 = (t-37*Tt/2)/Tt;
 t28 = (t-39*Tt/2)/Tt;
 t29 = (t-41*Tt/2)/Tt;
 t30 = (t-43*Tt/2)/(Tt/2);
 t31 = (t-44*Tt/2)/(Tt/2);
 t32 = (t-45*Tt/2)/Tt;
 t33 = (t-47*Tt/2)/(Tt/2);
 t34 = (t-48*Tt/2)/(Tt/2);
 t35 = (t-49*Tt/2)/Tt;
 t36 = (t-51*Tt/2)/(Tt/2);
 t37 = (t-52*Tt/2)/(Tt/2);
 t38 = (t-53*Tt/2)/Tt;
 t39 = (t-55*Tt/2)/Tt;
 t40 = (t-57*Tt/2)/Tt;
 t41 = (t-59*Tt/2)/(Tt/2);
 t42 = (t-60*Tt/2)/(Tt/2);
 t43 = (t-61*Tt/2)/Tt;
 t44 = (t-63*Tt/2)/(Tt/2);
 
 if t > 0 && t <= Tt/2 % 1
     [G, F] = ldm7t(t1);
     x = 0;
     x_p = 0;
     y = -G*l;
     y_p = -F*l/(Tt/2);
     
 elseif t > Tt/2 && t <= 3*Tt/2 % 2
     [G, F] = ldm7t(t2);
     x = G*3*l;
     x_p = F*3*l/Tt;
     y = -l;
     y_p = 0;
     
 elseif t > 3*Tt/2 && t <= 4*Tt/2 % 3
     [G, F] = ldm7t(t3);
     x = 3*l;
     x_p = 0;
     y = -l + G*l;
     y_p = F*l/(Tt/2);
     
  elseif t > 4*Tt/2 && t <= 5*Tt/2 % 4
     [G, F] = ldm7t(t4);
     x = 3*l - G*l;
     x_p = -F*l/(Tt/2);
     y = 0;
     y_p = 0;
     
  elseif t > 5*Tt/2 && t <= 7*Tt/2 % 5
     [G, F] = ldm7t(t5);
     x = 2*l;
     x_p = 0;
     y = -G*3*l;
     y_p = -F*3*l/Tt;
     
  elseif t > 7*Tt/2 && t <= 9*Tt/2 % 6
     [G, F] = ldm7t(t6);
     x = 2*l + G*3*l;
     x_p = F*3*l/Tt;
     y = -3*l;
     y_p = 0;
     
  elseif t > 9*Tt/2 && t <= 11*Tt/2 % 7
     [G, F] = ldm7t(t7);
     x = 5*l;
     x_p = 0;
     y = -3*l + G*3*l;
     y_p = -F*3*l/Tt;
     
   elseif t > 11*Tt/2 && t <= 12*Tt/2 % 8
     [G, F] = ldm7t(t8);
     x = 5*l - G*l;
     x_p = -F*l/(Tt/2);
     y = 0;
     y_p = 0;   
     
   elseif t > 12*Tt/2 && t <= 13*Tt/2 % 9
     [G, F] = ldm7t(t9);
     x = 4*l;
     x_p = 0;
     y = -G*l;
     y_p = -F*l/(Tt/2);   
     
   elseif t > 13*Tt/2 && t <= 15*Tt/2 % 10
     [G, F] = ldm7t(t10);
     x = 4*l + G*3*l;
     x_p = F*3*l/Tt;
     y = -l;
     y_p = 0;
     
   elseif t > 15*Tt/2 && t <= 16*Tt/2 % 11
     [G, F] = ldm7t(t11);
     x = 7*l;
     x_p = 0;
     y = -l + G*l;
     y_p = F*l/(Tt/2);
     
   elseif t > 16*Tt/2 && t <= 17*Tt/2 % 12
     [G, F] = ldm7t(t12);
     x = 7*l - G*l;
     x_p = -F*l/(Tt/2);
     y = 0;
     y_p = 0;
     
   elseif t > 17*Tt/2 && t <= 19*Tt/2 % 13
     [G, F] = ldm7t(t13);
     x = 6*l;
     x_p = 0;
     y = -G*3*l;
     y_p = -F*3*l/Tt;
     
   elseif t > 19*Tt/2 && t <= 20*Tt/2 % 14
     [G, F] = ldm7t(t14);
     x = 6*l + G*l;
     x_p = F*l/(Tt/2);
     y = -3*l;
     y_p = 0;
     
   elseif t > 20*Tt/2 && t <= 21*Tt/2 % 15
     [G, F] = ldm7t(t15);
     x = 7*l;
     x_p = 0;
     y = -3*l + G*l;
     y_p = F*l/(Tt/2);
     
   elseif t > 21*Tt/2 && t <= 23*Tt/2 % 16
     [G, F] = ldm7t(t16);
     x = 7*l - G*3*l;
     x_p = -F*3*l/Tt;
     y = -2*l;
     y_p = 0;
     
   elseif t > 23*Tt/2 && t <= 25*Tt/2 % 17
     [G, F] = ldm7t(t17);
     x = 4*l;
     x_p = 0;
     y = -2*l - 3*G*l;
     y_p = -F*3*l/Tt;
     
   elseif t > 25*Tt/2 && t <= 27*Tt/2 % 18
     [G, F] = ldm7t(t18);
     x = 4*l + 3*G*l;
     x_p = F*3*l/Tt;
     y = -5*l;
     y_p = 0;
     
   elseif t > 27*Tt/2 && t <= 28*Tt/2 % 19
     [G, F] = ldm7t(t19);
     x = 7*l;
     x_p = 0;
     y = -5*l + G*l;
     y_p = F*l/(Tt/2);
     
   elseif t > 28*Tt/2 && t <= 29*Tt/2 % 20
     [G, F] = ldm7t(t20);
     x = 7*l - G*l;
     x_p = -F*l/(Tt/2);
     y = -4*l;
     y_p = 0;
     
   elseif t > 29*Tt/2 && t <= 31*Tt/2 % 21
     [G, F] = ldm7t(t21);
     x = 6*l;
     x_p = 0;
     y = -4*l - 3*G*l;
     y_p = -F*3*l/Tt;
     
   elseif t > 31*Tt/2 && t <= 32*Tt/2 % 22
     [G, F] = ldm7t(t22);
     x = 6*l + G*l;
     x_p = F*l/(Tt/2);
     y = -7*l;
     y_p = 0;
     
   elseif t > 32*Tt/2 && t <= 33*Tt/2 % 23
     [G, F] = ldm7t(t23);
     x = 7*l;
     x_p = 0;
     y = -7*l + G*l;
     y_p = F*l/(Tt/2);
     
   elseif t > 33*Tt/2 && t <= 35*Tt/2 % 24
     [G, F] = ldm7t(t24);
     x = 7*l - 3*G*l;
     x_p = -F*3*l/Tt;
     y = -6*l;
     y_p = 0;
     
   elseif t > 35*Tt/2 && t <= 36*Tt/2 % 25
     [G, F] = ldm7t(t25);
     x = 4*l;
     x_p = 0;
     y = -6*l - G*l;
     y_p = -F*l/(Tt/2);
     
   elseif t > 36*Tt/2 && t <= 37*Tt/2 % 26
     [G, F] = ldm7t(t26);
     x = 4*l + G*l;
     x_p = F*l/(Tt/2);
     y = -7*l;
     y_p = 0;
     
   elseif t > 37*Tt/2 && t <= 39*Tt/2 % 27
     [G, F] = ldm7t(t27);
     x = 5*l;
     x_p = 0;
     y = -7*l + 3*G*l;
     y_p = F*3*l/Tt;
     
   elseif t > 39*Tt/2 && t <= 41*Tt/2 % 28
     [G, F] = ldm7t(t28);
     x = 5*l - 3*G*l;
     x_p = -F*3*l/Tt;
     y = -4*l;
     y_p = 0;
     
   elseif t > 41*Tt/2 && t <= 43*Tt/2 % 29
     [G, F] = ldm7t(t29);
     x = 2*l;
     x_p = 0;
     y = -4*l - G*3*l;
     y_p = -F*3*l/Tt;
     
   elseif t > 43*Tt/2 && t <= 44*Tt/2 % 30
     [G, F] = ldm7t(t30);
     x = 2*l + G*l;
     x_p = F*l/(Tt/2);
     y = -7*l;
     y_p = 0;
     
   elseif t > 44*Tt/2 && t <= 45*Tt/2 % 31
     [G, F] = ldm7t(t31);
     x = 3*l;
     x_p = 0;
     y = -7*l + G*l;
     y_p = F*l/(Tt/2);
     
   elseif t > 45*Tt/2 && t <= 47*Tt/2 % 32
     [G, F] = ldm7t(t32);
     x = 3*l - 3*G*l;
     x_p = -F*3*l/Tt;
     y = -6*l;
     y_p = 0;
     
   elseif t > 47*Tt/2 && t <= 48*Tt/2 % 33
     [G, F] = ldm7t(t33);
     x = 0;
     x_p = 0;
     y = -6*l - G*l;
     y_p = -F*l/(Tt/2);
     
   elseif t > 48*Tt/2 && t <= 49*Tt/2 % 34
     [G, F] = ldm7t(t34);
     x = G*l;
     x_p = F*l/(Tt/2);
     y = -7*l;
     y_p = 0;
     
   elseif t > 49*Tt/2 && t <= 51*Tt/2 % 35
     [G, F] = ldm7t(t35);
     x = l;
     x_p = 0;
     y = -7*l + 3*G*l;
     y_p = F*3*l/Tt;
     
   elseif t > 51*Tt/2 && t <= 52*Tt/2 % 36
     [G, F] = ldm7t(t36);
     x = l - G*l;
     x_p = -F*l/(Tt/2);
     y = -4*l;
     y_p = 0;
     
   elseif t > 52*Tt/2 && t <= 53*Tt/2 % 37
     [G, F] = ldm7t(t37);
     x = 0;
     x_p = 0;
     y = -4*l - G*l;
     y_p = -F*l/(Tt/2);
     
   elseif t > 53*Tt/2 && t <= 55*Tt/2 % 38
     [G, F] = ldm7t(t38);
     x = 3*G*l;
     x_p = F*3*l/Tt;
     y = -5*l;
     y_p = 0;
     
   elseif t > 55*Tt/2 && t <= 57*Tt/2 % 39
     [G, F] = ldm7t(t39);
     x = 3*l;
     x_p = 0;
     y = -5*l + G*3*l;
     y_p = F*3*l/Tt;
     
   elseif t > 57*Tt/2 && t <= 59*Tt/2 % 40
     [G, F] = ldm7t(t40);
     x = 3*l -G*3*l;
     x_p = -F*3*l/Tt;
     y = -2*l;
     y_p = 0;
     
   elseif t > 59*Tt/2 && t <= 60*Tt/2 % 41
     [G, F] = ldm7t(t41);
     x = 0;
     x_p = 0;
     y = -2*l - G*l;
     y_p = -F*l/(Tt/2);
     
   elseif t > 60*Tt/2 && t <= 61*Tt/2 % 42
     [G, F] = ldm7t(t42);
     x = G*l;
     x_p = F*l/(Tt/2);
     y = -3*l;
     y_p = 0;
     
   elseif t > 61*Tt/2 && t <= 63*Tt/2 % 43
     [G, F] = ldm7t(t43);
     x = l;
     x_p = 0;
     y = -3*l + 3*G*l;
     y_p = F*3*l/Tt;
     
   elseif t > 63*Tt/2 && t <= 64*Tt/2 % 44
     [G, F] = ldm7t(t44);
     x = l - G*l;
     x_p = -F*l/(Tt/2);
     y = 0;
     y_p = 0;
     
 else
     x = 0;
     x_p = 0;
     y = 0;
     y_p = 0;
 end

== matlab function State_Flow_D/Movimento Braccia/Subsystem/Cerchi Tangenti ==
  data: xct output; t input; yct output; d input; xct_p output; yct_p output
function [xct, yct, xct_p, yct_p] = fcn(t, d)

d1 = d;
T1 = 100*d1/2;
d2 = d1-0.025;
T2 = 100*d2/2;
d3 = d2-0.025;
T3 = 100*d3/2;
d4 = d3-0.025;
T4 = 100*d4/2;
d5 = d4-0.025;
T5 = 100*d5/2;

 t1 = (t)/(T1);
 t2 = (t-T1)/(T2);
 t3 = (t-T1-T2)/(T3);
 t4 = (t-T1-T2-T3)/(T4);
 t5 = (t-T1-T2-T3-T4)/(T5);

  if t > 0 && t <= T1 % 1
     [G, F] = ldm7t(t1);
     alfa = G*2*pi;
     alfa_p = F*2*pi/T1;
     xct = d1/2*cos(pi/2-alfa);
     yct = d1/2*sin(pi/2-alfa) - d1/2;
     xct_p = d1/2*sin(pi/2-alfa)*alfa_p;
     yct_p = -d1/2*cos(pi/2-alfa)*alfa_p;
     
 elseif t > T1 && t <= (T1+T2) % 2
     [G, F] = ldm7t(t2);
     alfa = G*2*pi;
     alfa_p = F*2*pi/T2;
     xct = d2/2*cos(pi/2-alfa);
     yct = d2/2*sin(pi/2-alfa) - d2/2;
     xct_p = d2/2*sin(pi/2-alfa)*alfa_p;
     yct_p = -d2/2*cos(pi/2-alfa)*alfa_p;
     
elseif t > (T1+T2) && t <= (T1+T2+T3) % 3
     [G, F] = ldm7t(t3);
     alfa = G*2*pi;
     alfa_p = F*2*pi/T3;
     xct = d3/2*cos(pi/2-alfa);
     yct = d3/2*sin(pi/2-alfa) - d3/2;
     xct_p = d3/2*sin(pi/2-alfa)*alfa_p;
     yct_p = -d3/2*cos(pi/2-alfa)*alfa_p;
     
elseif t > (T1+T2+T3) && t <= (T1+T2+T3+T4) % 4
     [G, F] = ldm7t(t4);
     alfa = G*2*pi;
     alfa_p = F*2*pi/T4;
     xct = d4/2*cos(pi/2-alfa);
     yct = d4/2*sin(pi/2-alfa) - d4/2;
     xct_p = d4/2*sin(pi/2-alfa)*alfa_p;
     yct_p = -d4/2*cos(pi/2-alfa)*alfa_p;
     
elseif t > (T1+T2+T3+T4) && t <= (T1+T2+T3+T4+T5) % 5
     [G, F] = ldm7t(t5);
     alfa = G*2*pi;
     alfa_p = F*2*pi/T5;
     xct = d5/2*cos(pi/2-alfa);
     yct = d5/2*sin(pi/2-alfa) - d5/2;
     xct_p = d5/2*sin(pi/2-alfa)*alfa_p;
     yct_p = -d5/2*cos(pi/2-alfa)*alfa_p;
 else
     xct = 0;
     xct_p = 0;
     yct = 0;
     yct_p = 0;
 end

== matlab function State_Flow_D/Movimento Braccia/Subsystem/spirale ==
  data: xs output; t input; ys output; T input; xs_p output; ys_p output; Rmax input; N input; Rmin input; T1 input
function [xs, ys, xs_p, ys_p] = fcn(t, T, Rmax, N, Rmin, T1)

t1 = t/T1;
t2 = (t-T1)/T;
if t >= 0 && t <= T1
    [G, F] = ldm7t(t1);
     xs = G*Rmin;
     xs_p = F*Rmin/T1;
     ys = 0;
     ys_p = 0;
elseif t > T1 && t <= T1+T 
    [G, F] = ldm7t(t2);
    r = Rmin + G*Rmax;
    r_p = F*Rmax/T;
    alfa = G*N*2*pi;
    alfa_p = F*N*2*pi/T;
    xs = r*cos(alfa);
    ys = r*sin(alfa);
    xs_p = -r*sin(alfa)*alfa_p + r_p*cos(alfa);
    ys_p = r*cos(alfa)*alfa_p + r_p*sin(alfa);
else
     xs = (Rmin+Rmax)*cos(N*2*pi);
     xs_p = 0;
     ys = (Rmin+Rmax)*sin(N*2*pi);
     ys_p = 0;
 end

== matlab function State_Flow_D/Movimento Braccia/MATLAB Function1 ==
  data: x input; xp output; z input; zp output; bool input
function [xp,zp] = fcn(x, z, bool)
if bool == 4
    xp = x;
    zp = -z;
else
    xp = 0;
    zp = 0;
end

== matlab function State_Flow_D/Movimento/Cinematica diretta ==
  data: x output; theta1 input; y output; theta2 input
function [x, y] = fcn(theta1, theta2)
d = 0.09;
l = 0.25;


A = l^2*(sin(theta2)-sin(theta1))^2 + (-2*d -l*(cos(theta2)-cos(theta1)))^2;
B = -2*l^2*d*(sin(theta2)-sin(theta1))*(cos(theta2)+cos(theta1)) + ...
    l*(sin(theta2)-sin(theta1))*(-2*d -l*(cos(theta2)-cos(theta1)))*(-2*d -2*l*cos(theta2)) - ...
    2*l*sin(theta2)*(-2*d -l*(cos(theta2)-cos(theta1)))^2;
C = l^2*d^2*(cos(theta2)+cos(theta1))^2 -l*d*(cos(theta2)+cos(theta1))*(-2*d -l*(cos(theta2)-cos(theta1)))*(-2*d -2*l*cos(theta2)) + ...
    (d^2 + 2*d*l*cos(theta2))*(-2*d - l*(cos(theta2)-cos(theta1)))^2;

% Posizione Y end-effector
y = (-B + sqrt(B^2 - 4*A*C))/(2*A);
% Posizione X end-effector
x = (y*l*(sin(theta2)-sin(theta1)) - l*d*(cos(theta2)+cos(theta1)))/(-2*d -l*(cos(theta2)-cos(theta1)));

== matlab function State_Flow_D/Movimento/Pos iniziali/Cinematica Inversa2 ==
  data: theta1_0 input; theta2_0 input; x0 output; y0 output
function [x0, y0] = fcn(theta1_0, theta2_0)

d = 0.09; 
l = 0.25;

A = l^2*(sin(theta2_0)-sin(theta1_0))^2 + (-2*d -l*(cos(theta2_0)-cos(theta1_0)))^2;
B = -2*l^2*d*(sin(theta2_0)-sin(theta1_0))*(cos(theta2_0)+cos(theta1_0)) + ...
    l*(sin(theta2_0)-sin(theta1_0))*(-2*d -l*(cos(theta2_0)-cos(theta1_0)))*(-2*d -2*l*cos(theta2_0)) - ...
    2*l*sin(theta2_0)*(-2*d -l*(cos(theta2_0)-cos(theta1_0)))^2;
C = l^2*d^2*(cos(theta2_0)+cos(theta1_0))^2 -l*d*(cos(theta2_0)+cos(theta1_0))*(-2*d -l*(cos(theta2_0)-cos(theta1_0)))*(-2*d -2*l*cos(theta2_0)) + ...
    (d^2 + 2*d*l*cos(theta2_0))*(-2*d - l*(cos(theta2_0)-cos(theta1_0)))^2;

% Posizione Y end-effector
y0 = (-B + sqrt(B^2 - 4*A*C))/(2*A);
% Posizione X end-effector
x0 = (y0*l*(sin(theta2_0)-sin(theta1_0)) - l*d*(cos(theta2_0)+cos(theta1_0)))/(-2*d -l*(cos(theta2_0)-cos(theta1_0)));

== matlab function State_Flow_D/Movimento/MATLAB Function1 ==
  data: x input; xp output; z input; zp output; bool input
function [xp,zp] = fcn(x, z, bool)
if bool == 4
    xp = x;
    zp = -z;
else
    xp = 0;
    zp = 0;
end

== matlab function State_Flow_D/Movimento/Leggi di moto/Cerchi Tangenti ==
  data: xct output; t input; yct output; d input; xct_p output; yct_p output; xct_pp output; yct_pp output
function [xct, yct, xct_p, yct_p, xct_pp, yct_pp] = fcn(t, d)

d1 = d;
T1 = 100*d1/2;
d2 = d1-0.025;
T2 = 100*d2/2;
d3 = d2-0.025;
T3 = 100*d3/2;
d4 = d3-0.025;
T4 = 100*d4/2;
d5 = d4-0.025;
T5 = 100*d5/2;

 t1 = (t)/(T1);
 t2 = (t-T1)/(T2);
 t3 = (t-T1-T2)/(T3);
 t4 = (t-T1-T2-T3)/(T4);
 t5 = (t-T1-T2-T3-T4)/(T5);

  if t > 0 && t <= T1 % 1
     [G, F, f] = ldm7t(t1);
     alfa = G*2*pi;
     alfa_p = F*2*pi/T1;
     alfa_pp = f*2*pi/(T1^2);
     xct = d1/2*cos(pi/2-alfa);
     yct = d1/2*sin(pi/2-alfa) - d1/2;
     xct_p = d1/2*sin(pi/2-alfa)*alfa_p;
     yct_p = -d1/2*cos(pi/2-alfa)*alfa_p;
     xct_pp = -d1/2*cos(pi/2-alfa)*alfa_p^2 + d1/2*sin(pi/2-alfa)*alfa_pp;
     yct_pp = -d1/2*sin(pi/2-alfa)*alfa_p^2- d1/2*cos(pi/2-alfa)*alfa_pp;
     
 elseif t > T1 && t <= (T1+T2) % 2
     [G, F, f] = ldm7t(t2);
     alfa = G*2*pi;
     alfa_p = F*2*pi/T2;
     alfa_pp = f*2*pi/(T2^2);
     xct = d2/2*cos(pi/2-alfa);
     yct = d2/2*sin(pi/2-alfa) - d2/2;
     xct_p = d2/2*sin(pi/2-alfa)*alfa_p;
     yct_p = -d2/2*cos(pi/2-alfa)*alfa_p;
     xct_pp = -d2/2*cos(pi/2-alfa)*alfa_p^2 + d2/2*sin(pi/2-alfa)*alfa_pp;
     yct_pp = -d2/2*sin(pi/2-alfa)*alfa_p^2- d2/2*cos(pi/2-alfa)*alfa_pp;
     
elseif t > (T1+T2) && t <= (T1+T2+T3) % 3
     [G, F, f] = ldm7t(t3);
     alfa = G*2*pi;
     alfa_p = F*2*pi/T3;
     alfa_pp = f*2*pi/(T3^2);
     xct = d3/2*cos(pi/2-alfa);
     yct = d3/2*sin(pi/2-alfa) - d3/2;
     xct_p = d3/2*sin(pi/2-alfa)*alfa_p;
     yct_p = -d3/2*cos(pi/2-alfa)*alfa_p;
     xct_pp = -d3/2*cos(pi/2-alfa)*alfa_p^2 + d3/2*sin(pi/2-alfa)*alfa_pp;
     yct_pp = -d3/2*sin(pi/2-alfa)*alfa_p^2- d3/2*cos(pi/2-alfa)*alfa_pp;
     
elseif t > (T1+T2+T3) && t <= (T1+T2+T3+T4) % 4
     [G, F, f] = ldm7t(t4);
     alfa = G*2*pi;
     alfa_p = F*2*pi/T4;
     alfa_pp = f*2*pi/(T4^2);
     xct = d4/2*cos(pi/2-alfa);
     yct = d4/2*sin(pi/2-alfa) - d4/2;
     xct_p = d4/2*sin(pi/2-alfa)*alfa_p;
     yct_p = -d4/2*cos(pi/2-alfa)*alfa_p;
     xct_pp = -d4/2*cos(pi/2-alfa)*alfa_p^2 + d4/2*sin(pi/2-alfa)*alfa_pp;
     yct_pp = -d4/2*sin(pi/2-alfa)*alfa_p^2- d4/2*cos(pi/2-alfa)*alfa_pp;
     
elseif t > (T1+T2+T3+T4) && t <= (T1+T2+T3+T4+T5) % 5
     [G, F, f] = ldm7t(t5);
     alfa = G*2*pi;
     alfa_p = F*2*pi/T5;
     alfa_pp = f*2*pi/(T5^2);
     xct = d5/2*cos(pi/2-alfa);
     yct = d5/2*sin(pi/2-alfa) - d5/2;
     xct_p = d5/2*sin(pi/2-alfa)*alfa_p;
     yct_p = -d5/2*cos(pi/2-alfa)*alfa_p;
     xct_pp = -d5/2*cos(pi/2-alfa)*alfa_p^2 + d5/2*sin(pi/2-alfa)*alfa_pp;
     yct_pp = -d5/2*sin(pi/2-alfa)*alfa_p^2- d5/2*cos(pi/2-alfa)*alfa_pp;
 else
     xct = 0;
     xct_p = 0;
     yct = 0;
     yct_p = 0;
     xct_pp = 0;
     yct_pp = 0;
 end

== matlab function State_Flow_D/Movimento/Cinematica Inversa ==
  data: x input; theta1 output; y input; theta2 output
function [theta1, theta2] = fcn(x, y)

d = 0.09; 
l = 0.25;

p = 2*d*l + 2*x*l;
e = 2*y*l;
f = x^2 + d^2 + y^2 + 2*x*d;
a = -2*d*l + 2*x*l;
b = +2*y*l;
c = x^2 + d^2 + y^2 - 2*x*d;



   theta1 = 2*atan2(e + sqrt(p^2 + e^2 -f^2), p +f);


   theta2 = 2*atan2(b - sqrt(a^2 + b^2 -c^2), a +c);
   if (theta2) < -deg2rad(200)
       theta2 = theta2 + 2*pi;
   end

== matlab function State_Flow_D/Movimento/Cinematica Inversa vel ==
  data: theta1 input; theta2 input; x input; y input; xp input; theta1_p output; yp input; theta2_p output
function [theta1_p, theta2_p] = fcn(theta1, theta2,x, y, xp, yp)

d = 0.09; 
l = 0.25;

N21 = -l*sin(theta1)*(x+d-l*cos(theta1)) + l*cos(theta1)*(y-l*sin(theta1));

N22 = -l*cos(theta2)*(y-l*sin(theta2))*(x+d-l*cos(theta1))/(x-d-l*cos(theta2)) + l*sin(theta2)*(x+d-l*cos(theta1));

D2 = y-l*sin(theta1) - (y-l*sin(theta2))*(x+d-l*cos(theta1))/(x-d-l*cos(theta2));

J21 = N21/D2;

J22 = N22/D2;

J11 = -(y-l*sin(theta2))/(x-d-l*cos(theta2))*(J21);

J12 = -(y-l*sin(theta2))/(x-d-l*cos(theta2))*(J22) -l*sin(theta2) + (y-l*sin(theta2))/(x-d-l*cos(theta2))*(l*cos(theta2));

J = [J11 J12; J21 J22];

theta_p = J^-1 * [xp; yp];
theta1_p = theta_p(1);
theta2_p = theta_p(2);
